simulink model "continuous"  (R2017a)
settings: Solver=VariableStepAuto  StartTime=0.0  StopTime=20.0  RelTol=1e-3
settings Model: Creator=aous  LastModifiedBy=aous

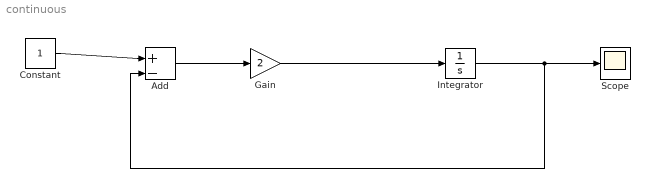
== system continuous ==
  Add : Sum  Inputs=+|-
  Constant : Constant
  Gain : Gain  Gain=2
  Integrator : Integrator
  Scope : Scope
  wires:
  Gain/1 -> Integrator/1
  Constant/1 -> Add/1
  Add/1 -> Gain/1
  Integrator/1 -> Scope/1, Add/2
